simulink model "HITL_Controller_top"  (R2024b)
settings: configuration reference "DeploymentConfiguration" (kept outside this file)
undefined symbols (not defined in the file): CityMission, control, FixedWingMission, HoverMission, TransitionMission
libraries: px4uORBlib x7, robotcorelib x3, px4Peripheralslib x1
settings Model: DataDictionary=VTOLDynamicsData.sldd  SimulationMode=external  ExtModeTrigDuration=10  Creator=The MathWorks, Inc.  LastModifiedBy=The MathWorks, Inc.
settings ConfigSetRef: SourceName=DeploymentConfiguration

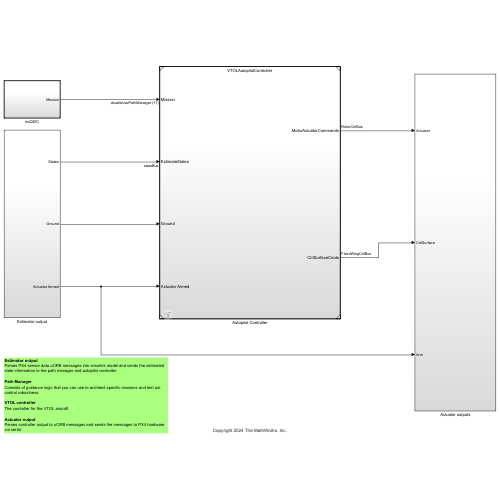
[thumbnail: Simulink's stored preview of the top-level diagram]
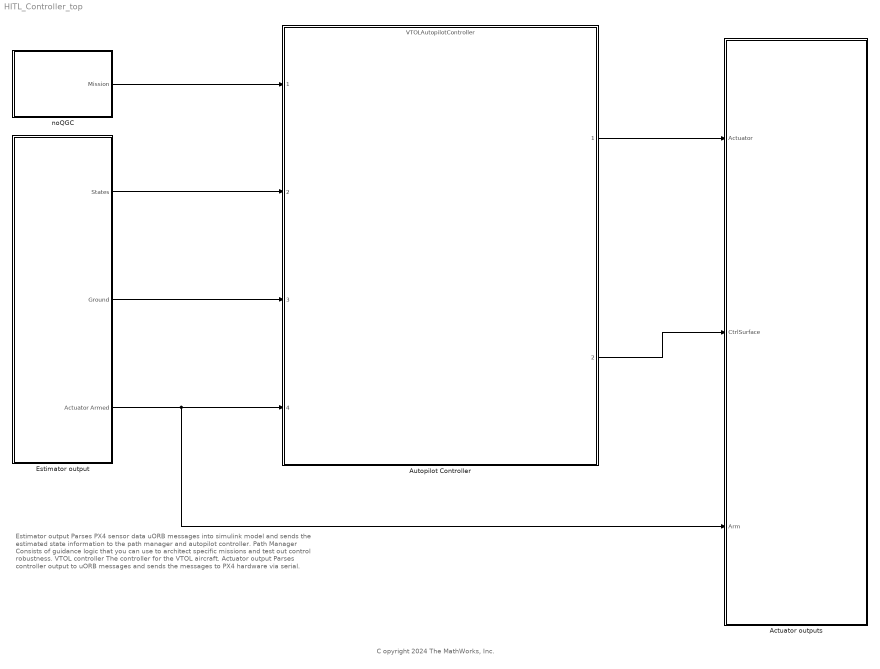
== system HITL_Controller_top ==
  note: Estimator output
      | Parses PX4 sensor data uORB messages into simulink model and sends the estimated state information to the path manager and autopilot controller.
      |
      | Path Manager
      | Consists of guidance logic that you can use to architect specific missions and test out control robustness.
      |
      | VTOL controller
      | The controller for the VTOL aircraft.
      |
      | Actuator output
      | Parses controller output to uORB messages and sends the messages to PX4 hardware via serial.
  note: C opyright 2024 The MathWorks, Inc.
  Actuator outputs : Subsystem
  Autopilot Controller : ModelReference  ModelNameDialog=VTOLAutopilotController  SimulationMode=Normal  ModelReferenceVersion=1.104
  Estimator output : Subsystem
  noQGC : Subsystem  TreatAsAtomicUnit=on  VariantControl=useQGC==0
  wires:
  noQGC/1(Mission) -> Autopilot Controller/1
  Estimator output/3(Actuator Armed) -> Actuator outputs/3(Arm), Autopilot Controller/4
  Estimator output/2(Ground) -> Autopilot Controller/3
  Estimator output/1(States) -> Autopilot Controller/2
  Autopilot Controller/1 -> Actuator outputs/1(Actuator)
  Autopilot Controller/2 -> Actuator outputs/2(CtrlSurface)

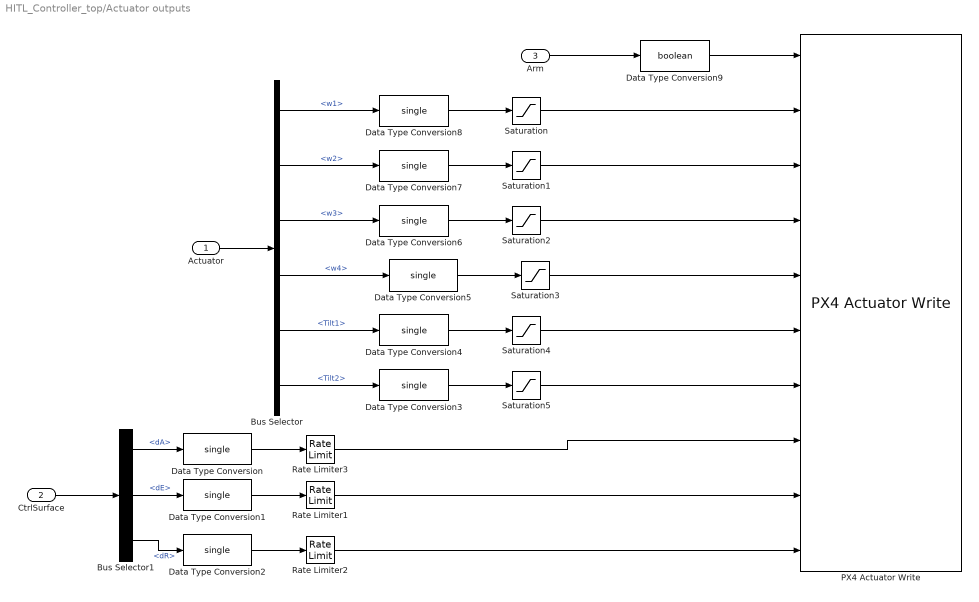
== system HITL_Controller_top/Actuator outputs ==
  Actuator : Inport
  CtrlSurface : Inport  Port=2
  Arm : Inport  Port=3
  Bus Selector : BusSelector  OutputSignals=w1,w2,w3,w4,Tilt1,Tilt2
  Bus Selector1 : BusSelector  OutputSignals=dA,dE,dR
  Data Type Conversion{,1..8} (9 alike) : DataTypeConversion  OutDataTypeStr=single  SaturateOnIntegerOverflow=off  RndMeth=Floor
  Data Type Conversion9 : DataTypeConversion  OutDataTypeStr=boolean  SaturateOnIntegerOverflow=off  RndMeth=Floor
  PX4 Actuator Write : px4Peripheralslib/PX4 Actuator Write  Motor1Enable=on  Motor2Enable=on  Motor3Enable=on  Motor4Enable=on  Motor5Enable=off  Motor6Enable=off  Motor7Enable=off  Motor8Enable=off  Motor9Enable=off  Motor10Enable=off  Motor11Enable=off  Motor12Enable=off  IsMotorArray=off  Servo1Enable=on  Servo2Enable=on  Servo3Enable=on  Servo4Enable=on  Servo5Enable=on  Servo6Enable=off  Servo7Enable=off  Servo8Enable=off  IsServoArray=off
  Rate Limiter1 : RateLimiter  RisingSlewLimit=control.slewRateServos  FallingSlewLimit=-control.slewRateServos  SampleTimeMode=inherited
  Rate Limiter2 : RateLimiter  RisingSlewLimit=control.slewRateServos  FallingSlewLimit=-control.slewRateServos  SampleTimeMode=inherited
  Rate Limiter3 : RateLimiter  RisingSlewLimit=control.slewRateServos  FallingSlewLimit=-control.slewRateServos  SampleTimeMode=inherited
  Saturation{,1..3} (4 alike) : Saturate  UpperLimit=single(0.9)  LowerLimit=0
  Saturation4 : Saturate  UpperLimit=single(1)  LowerLimit=single(-0.2)
  Saturation5 : Saturate  UpperLimit=single(1)  LowerLimit=single(-0.2)
  wires:
  Rate Limiter3/1 -> PX4 Actuator Write/8
  Bus Selector1/2 -> Data Type Conversion1/1  "<dE>"
  Rate Limiter2/1 -> PX4 Actuator Write/10
  Rate Limiter1/1 -> PX4 Actuator Write/9
  Bus Selector1/3 -> Data Type Conversion2/1  "<dR>"
  Bus Selector/4 -> Data Type Conversion5/1  "<w4>"
  Actuator/1 -> Bus Selector/1
  Bus Selector/2 -> Data Type Conversion7/1  "<w2>"
  Bus Selector/6 -> Data Type Conversion3/1  "<Tilt2>"
  Bus Selector/3 -> Data Type Conversion6/1  "<w3>"
  Bus Selector/1 -> Data Type Conversion8/1  "<w1>"
  Bus Selector1/1 -> Data Type Conversion/1  "<dA>"
  Bus Selector/5 -> Data Type Conversion4/1  "<Tilt1>"
  CtrlSurface/1 -> Bus Selector1/1
  Data Type Conversion/1 -> Rate Limiter3/1
  Data Type Conversion1/1 -> Rate Limiter1/1
  Data Type Conversion2/1 -> Rate Limiter2/1
  Data Type Conversion8/1 -> Saturation/1
  Data Type Conversion7/1 -> Saturation1/1
  Data Type Conversion6/1 -> Saturation2/1
  Data Type Conversion5/1 -> Saturation3/1
  Data Type Conversion4/1 -> Saturation4/1
  Data Type Conversion3/1 -> Saturation5/1
  Saturation/1 -> PX4 Actuator Write/2
  Saturation1/1 -> PX4 Actuator Write/3
  Saturation2/1 -> PX4 Actuator Write/4
  Saturation3/1 -> PX4 Actuator Write/5
  Saturation4/1 -> PX4 Actuator Write/6
  Saturation5/1 -> PX4 Actuator Write/7
  Arm/1 -> Data Type Conversion9/1
  Data Type Conversion9/1 -> PX4 Actuator Write/1

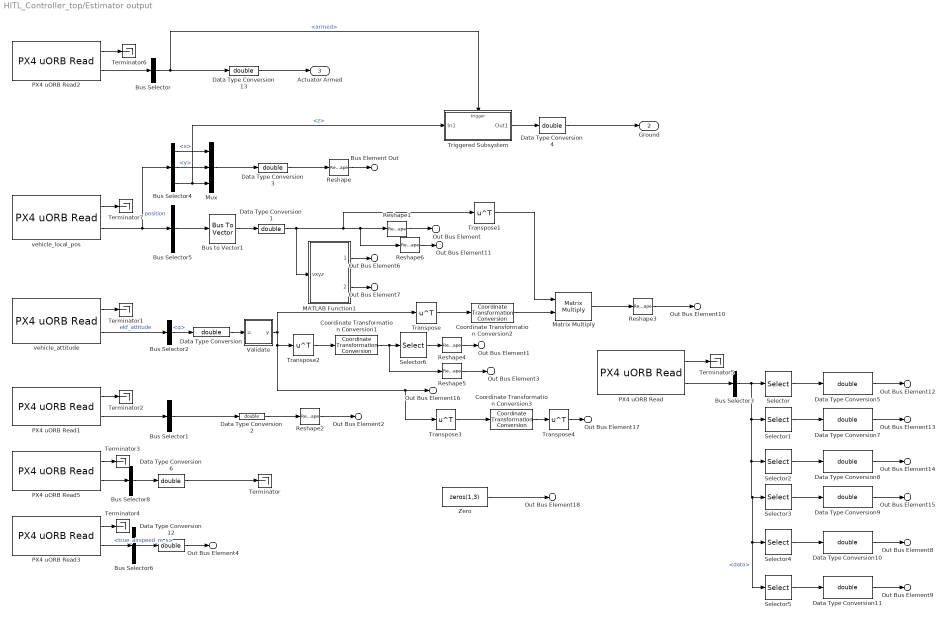
== system HITL_Controller_top/Estimator output ==
  Bus Selector : BusSelector  OutputSignals=armed
  Bus Selector1 : BusSelector  OutputSignals=angular_velocity  OutputAsBus=on
  Bus Selector2 : BusSelector  OutputSignals=q
  Bus Selector3 : BusSelector  OutputSignals=data
  Bus Selector4 : BusSelector  OutputSignals=x,y,z
  Bus Selector5 : BusSelector  OutputSignals=vx,vy,vz  OutputAsBus=on
  Bus Selector6 : BusSelector  OutputSignals=true_airspeed_m_s
  Bus Selector8 : BusSelector  OutputSignals=ground_contact  OutputAsBus=on
  Bus to Vector1 : BusToVector
  Coordinate Transformation Conversion1 : robotcorelib/Coordinate Transformation Conversion  InputRepresentation=Quaternion  InputEulerSequence=ZYX  ShowTrVecInputPort=on  OutputRepresentation=Euler Angles  OutputEulerSequence=ZYX  ShowTrVecOutputPort=on  SimulateUsing=Interpreted execution
      settings: LibrarySourceBlock=navlib/Utilities/Coordinate Transformation Conversion
  Coordinate Transformation Conversion2 : robotcorelib/Coordinate Transformation Conversion  InputRepresentation=Quaternion  InputEulerSequence=ZYX  ShowTrVecInputPort=on  OutputRepresentation=Rotation Matrix  OutputEulerSequence=ZYX  ShowTrVecOutputPort=on  SimulateUsing=Interpreted execution
      settings: LibrarySourceBlock=navlib/Utilities/Coordinate Transformation Conversion
  Coordinate Transformation Conversion3 : robotcorelib/Coordinate Transformation Conversion  InputRepresentation=Quaternion  InputEulerSequence=ZYX  ShowTrVecInputPort=on  OutputRepresentation=Rotation Matrix  OutputEulerSequence=ZYX  ShowTrVecOutputPort=on  SimulateUsing=Code generation
      settings: LibrarySourceBlock=navlib/Utilities/Coordinate Transformation Conversion
  Data Type Conversion{,1..13} (14 alike) : DataTypeConversion  OutDataTypeStr=double  SaturateOnIntegerOverflow=off  RndMeth=Floor
  MATLAB Function1 : MATLAB Function  TreatAsAtomicUnit=on
  Matrix Multiply : Product  Multiplication=Matrix(*)
  Mux : Mux  Inputs=3
  PX4 uORB Read : px4uORBlib/PX4 uORB Read  uORBTopic=DebugArray  selectInstance=DebugArray  SampleTime=-1  BlockingMode=off  BlockTimeout=1e-3
  PX4 uORB Read1 : px4uORBlib/PX4 uORB Read  uORBTopic=VehicleOdometry  selectInstance=vehicle_odometry  SampleTime=-1  BlockingMode=off  BlockTimeout=1e-3
  PX4 uORB Read2 : px4uORBlib/PX4 uORB Read  uORBTopic=ActuatorArmed  selectInstance=ActuatorArmed  SampleTime=-1  BlockingMode=off  BlockTimeout=1e-3
  PX4 uORB Read3 : px4uORBlib/PX4 uORB Read  uORBTopic=Airspeed  selectInstance=Airspeed  SampleTime=-1  BlockingMode=off  BlockTimeout=1e-3
  PX4 uORB Read5 : px4uORBlib/PX4 uORB Read  uORBTopic=VehicleLandDetected  selectInstance=VehicleLandDetected  SampleTime=-1  BlockingMode=off  BlockTimeout=1e-3
  Reshape{,1..2,4..6} (6 alike) : Reshape  OutputDimensionality=Column vector (2-D)
  Reshape3 : Reshape  OutputDimensionality=Row vector (2-D)
  Selector : Selector  InputPortWidth=58  IndexOptions=Index vector (dialog)  Indices=1  OutputSizes=1
  Selector1 : Selector  InputPortWidth=58  IndexOptions=Index vector (dialog)  Indices=2  OutputSizes=1
  Selector2 : Selector  InputPortWidth=58  IndexOptions=Index vector (dialog)  Indices=3  OutputSizes=1
  Selector3 : Selector  InputPortWidth=58  IndexOptions=Index vector (dialog)  Indices=4  OutputSizes=1
  Selector4 : Selector  InputPortWidth=58  IndexOptions=Index vector (dialog)  Indices=5  OutputSizes=1
  Selector5 : Selector  InputPortWidth=58  IndexOptions=Index vector (dialog)  Indices=6  OutputSizes=1
  Selector6 : Selector  InputPortWidth=3  IndexOptions=Index vector (dialog)  Indices=[3 2 1]  OutputSizes=1
  Terminator{,1..7} (8 alike) : Terminator
  Transpose{,1..4} (5 alike) : Math  Operator=transpose
  Triggered Subsystem : Subsystem  TreatAsAtomicUnit=on
  Validate : MATLAB Function  TreatAsAtomicUnit=on
  Zero : Constant  Value=zeros(1,3)  VectorParams1D=off  OutDataTypeStr=Inherit: Inherit via back propagation
  vehicle_attitude : px4uORBlib/PX4 uORB Read  uORBTopic=VehicleAttitude  selectInstance=vehicle_attitude  SampleTime=-1  BlockingMode=off  BlockTimeout=1e-3
  vehicle_local_pos : px4uORBlib/PX4 uORB Read  uORBTopic=VehicleLocalPosition  selectInstance=vehicle_local_position  SampleTime=-1  BlockingMode=off  BlockTimeout=1e-3
  Out Bus Element6 : Outport  PortName=States  Element=course
  Out Bus Element7 : Outport  PortName=States  Element=gndspeed
  Out Bus Element4 : Outport  PortName=States  Element=airspeed
  Bus Element Out : Outport  PortName=States  Element=Xe
  Out Bus Element : Outport  PortName=States  Element=Ve
  Out Bus Element17 : Outport  PortName=States  Element=DCMbe
  Out Bus Element16 : Outport  PortName=States  Element=q
  Out Bus Element2 : Outport  PortName=States  Element=pqr
  Out Bus Element10 : Outport  PortName=States  Element=Vb
  Out Bus Element18 : Outport  PortName=States  Element=Abb
  Out Bus Element1 : Outport  PortName=States  Element=Euler
  Out Bus Element12 : Outport  PortName=States  Element=RotorParameters.w1
  Out Bus Element13 : Outport  PortName=States  Element=RotorParameters.w2
  Out Bus Element14 : Outport  PortName=States  Element=RotorParameters.w3
  Out Bus Element15 : Outport  PortName=States  Element=RotorParameters.w4
  Out Bus Element8 : Outport  PortName=States  Element=RotorParameters.Tilt1
  Out Bus Element9 : Outport  PortName=States  Element=RotorParameters.Tilt2
  Out Bus Element3 : Outport  PortName=States  Element=ypr
  Out Bus Element11 : Outport  PortName=States  Element=Ve_ground
  Ground : Outport  Port=2
  Actuator Armed : Outport  Port=3
  wires:
  PX4 uORB Read2/2 -> Bus Selector/1
  Data Type Conversion/1 -> Validate/1(u)
  Data Type Conversion1/1 -> Transpose1/1, Reshape6/1, Reshape1/1, MATLAB Function1/1(vxyz)
  Data Type Conversion3/1 -> Reshape/1
  PX4 uORB Read5/2 -> Bus Selector8/1
  Bus Selector8/1 -> Data Type Conversion6/1
  PX4 uORB Read3/2 -> Bus Selector6/1
  Transpose1/1 -> Matrix Multiply/1
  vehicle_attitude/1 -> Terminator1/1
  vehicle_attitude/2 -> Bus Selector2/1  "ekf_attitude"
  Data Type Conversion2/1 -> Reshape2/1
  Mux/1 -> Data Type Conversion3/1
  PX4 uORB Read1/2 -> Bus Selector1/1
  Bus to Vector1/1 -> Data Type Conversion1/1
  MATLAB Function1/2(gndSpeed) -> Out Bus Element7/1
  vehicle_local_pos/2 -> Bus Selector4/1, Bus Selector5/1  "position"
  Transpose/1 -> Coordinate Transformation Conversion2/1
  PX4 uORB Read2/1 -> Terminator6/1
  Bus Selector4/3 -> Triggered Subsystem/1(In1), Mux/3  "<z>"
  Matrix Multiply/1 -> Reshape3/1
  Bus Selector2/1 -> Data Type Conversion/1  "<q>"
  MATLAB Function1/1(course) -> Out Bus Element6/1
  Bus Selector4/2 -> Mux/2  "<y>"
  Bus Selector/1 -> Data Type Conversion13/1, Triggered Subsystem/Trigger  "<armed>"
  PX4 uORB Read5/1 -> Terminator3/1
  Bus Selector5/1 -> Bus to Vector1/1
  Bus Selector4/1 -> Mux/1  "<x>"
  PX4 uORB Read1/1 -> Terminator2/1
  Data Type Conversion6/1 -> Terminator/1
  Validate/1(y) -> Transpose2/1, Transpose3/1, Out Bus Element16/1, Transpose/1
  Bus Selector1/1 -> Data Type Conversion2/1
  PX4 uORB Read3/1 -> Terminator4/1
  Coordinate Transformation Conversion2/1 -> Matrix Multiply/2
  Transpose2/1 -> Coordinate Transformation Conversion1/1
  PX4 uORB Read/2 -> Bus Selector3/1
  PX4 uORB Read/1 -> Terminator5/1
  Selector/1 -> Data Type Conversion5/1
  Bus Selector3/1 -> Selector5/1, Selector4/1, Selector3/1, Selector2/1, Selector1/1, Selector/1  "<data>"
  Selector1/1 -> Data Type Conversion7/1
  Selector2/1 -> Data Type Conversion8/1
  Selector3/1 -> Data Type Conversion9/1
  Selector4/1 -> Data Type Conversion10/1
  Selector5/1 -> Data Type Conversion11/1
  Data Type Conversion5/1 -> Out Bus Element12/1
  Data Type Conversion7/1 -> Out Bus Element13/1
  Data Type Conversion8/1 -> Out Bus Element14/1
  Data Type Conversion9/1 -> Out Bus Element15/1
  Data Type Conversion10/1 -> Out Bus Element8/1
  Data Type Conversion11/1 -> Out Bus Element9/1
  Coordinate Transformation Conversion1/1 -> Reshape5/1, Selector6/1
  Reshape2/1 -> Out Bus Element2/1
  Bus Selector6/1 -> Data Type Conversion12/1  "<true_airspeed_m_s>"
  Selector6/1 -> Reshape4/1
  Triggered Subsystem/1(Out1) -> Data Type Conversion4/1
  Data Type Conversion4/1 -> Ground/1
  vehicle_local_pos/1 -> Terminator7/1
  Coordinate Transformation Conversion3/1 -> Transpose4/1
  Transpose4/1 -> Out Bus Element17/1
  Zero/1 -> Out Bus Element18/1
  Reshape/1 -> Bus Element Out/1
  Reshape1/1 -> Out Bus Element/1
  Reshape3/1 -> Out Bus Element10/1
  Reshape4/1 -> Out Bus Element1/1
  Reshape5/1 -> Out Bus Element3/1
  Reshape6/1 -> Out Bus Element11/1
  Data Type Conversion12/1 -> Out Bus Element4/1
  Data Type Conversion13/1 -> Actuator Armed/1
  Transpose3/1 -> Coordinate Transformation Conversion3/1

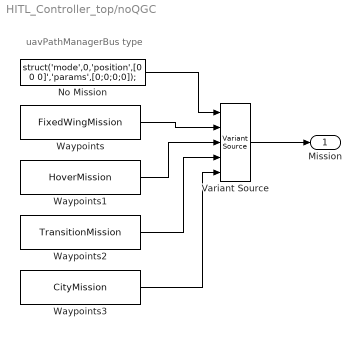
== system HITL_Controller_top/noQGC ==
  note: uavPathManagerBus type
  No Mission : Constant  Value=struct('mode',0,'position',[0 0 0]','params',[0;0;0;0]);  OutDataTypeStr=Bus: doubleUavPathManager
  Variant Source : VariantSource
  Waypoints : Constant  Value=FixedWingMission  OutDataTypeStr=Bus: doubleUavPathManager  SampleTime=-1
  Waypoints1 : Constant  Value=HoverMission  OutDataTypeStr=Bus: doubleUavPathManager  SampleTime=-1
  Waypoints2 : Constant  Value=TransitionMission  OutDataTypeStr=Bus: doubleUavPathManager  SampleTime=-1
  Waypoints3 : Constant  Value=CityMission  OutDataTypeStr=Bus: doubleUavPathManager  SampleTime=-1
  Mission : Outport
  wires:
  Waypoints/1 -> Variant Source/2
  Waypoints1/1 -> Variant Source/3
  Variant Source/1 -> Mission/1
  Waypoints2/1 -> Variant Source/4
  No Mission/1 -> Variant Source/1
  Waypoints3/1 -> Variant Source/5

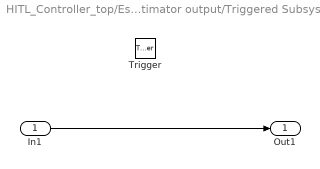
== system HITL_Controller_top/Estimator output/Triggered Subsystem ==
  In1 : Inport
  Trigger : TriggerPort  VariantControl=(inherit)
  Out1 : Outport
  wires:
  In1/1 -> Out1/1

== matlab function HITL_Controller_top/Estimator output/Validate ==
  data: u input; y output
function y = fcn(u)

if any(isnan(u))
    y = [1 0 0 0];
elseif norm(u)<0.1
    y = [1 0 0 0];
else
    y = u/norm(u);
end

end

== matlab function HITL_Controller_top/Estimator output/MATLAB Function1 ==
  data: vxyz input; course output; gndSpeed output
function [course, gndSpeed] = fcn(vxyz)

vx = vxyz(1);
vy = vxyz(2);

course = atan2(vy, vx);
gndSpeed = norm([vx, vy]);
